simulink model "flexibleBeamSim"  (R2019b)
settings: Solver=ode4  StartTime=0.0  StopTime=tin(end)  FixedStep=Ts  RelTol=1e-3
values from neighbouring files (symbols this model uses):
  shapeit_data =     [GyGzcontroller.mat]    (also in GyGzcontrollerBad.mat; GyGzcontrollerGood.mat; GyGzcontrollerWorse.mat; GzController5Hz.mat)
libraries: cstblocks x1
settings Model: Creator=maxva  LastModifiedBy=maxva

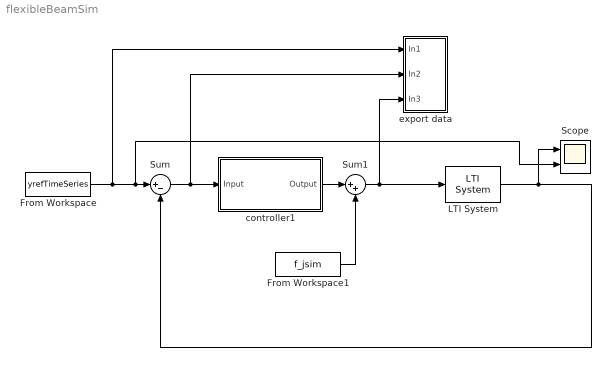
== system flexibleBeamSim ==
  From Workspace : FromWorkspace  VariableName=yrefTimeSeries  SampleTime=0
  From Workspace1 : FromWorkspace  VariableName=f_jsim  SampleTime=0
  LTI System : cstblocks/LTI System  sys=G  IC=[]
  Scope : Scope  NumInputPorts=2
  Sum : Sum  Inputs=|+-
  Sum1 : Sum  Inputs=|++
  controller1 : Subsystem
  export data : Subsystem
  wires:
  LTI System/1 -> Scope/1, Sum/2
  Sum1/1 -> LTI System/1, export data/3(In3)
  From Workspace/1 -> Scope/2, Sum/1, export data/1(In1)
  From Workspace1/1 -> Sum1/2
  Sum/1 -> controller1/1(Input), export data/2(In2)
  controller1/1(Output) -> Sum1/1

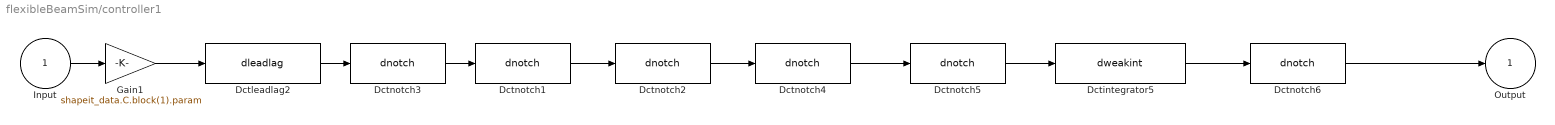
== system flexibleBeamSim/controller1 ==
  Input : Inport
  Dctintegrator5 : S-Function  FunctionName=dweakint  Parameters=f_num, 0.001  SFunctionDeploymentMode=off  EnableBusSupport=off  mask(dctools){f_num=shapeit_data.C.block(8).param}
      mask prompts: f_num "Zero [Hz]"
      mask help: This block implements a discrete time weak integrator filter.
      mask Display: disp('DCT integrator')
  Dctleadlag2 : S-Function  FunctionName=dleadlag  Parameters=f_num, f_den, 0.001  SFunctionDeploymentMode=off  EnableBusSupport=off  mask(dctools){f_num=shapeit_data.C.block(2).param(1), f_den=shapeit_data.C.block(2).param(2)}
      mask prompts: f_num "Zero [Hz]"; f_den "Pole [Hz]"
      mask help: This block implements a discrete time leadlag filter.
      mask Display: disp('DCT leadlag')
  Dctnotch1 : S-Function  FunctionName=dnotch  Parameters=f_num, b_num, f_den, b_den, 0.001  SFunctionDeploymentMode=off  EnableBusSupport=off  mask(dctools){f_num=shapeit_data.C.block(4).param(1), b_num=shapeit_data.C.block(4).param(2), f_den=shapeit_data.C.block(4).param(3), b_den=shapeit_data.C.block(4).param(4)}
      mask prompts: f_num "Zero [Hz]"; b_num "Damping zero [-]"; f_den "Pole [Hz]"; b_den "Damping pole [-]"
      mask help: This block implements a dicrete time 2nd order notch filter.
      mask Display: disp('DCT notch')
  Dctnotch2 : S-Function  FunctionName=dnotch  Parameters=f_num, b_num, f_den, b_den, 0.001  SFunctionDeploymentMode=off  EnableBusSupport=off  mask(dctools){f_num=shapeit_data.C.block(7).param(1), b_num=shapeit_data.C.block(7).param(2), f_den=shapeit_data.C.block(7).param(3), b_den=shapeit_data.C.block(7).param(4)}
      mask prompts: f_num "Zero [Hz]"; b_num "Damping zero [-]"; f_den "Pole [Hz]"; b_den "Damping pole [-]"
      mask help: This block implements a dicrete time 2nd order notch filter.
      mask Display: disp('DCT notch')
  Dctnotch3 : S-Function  FunctionName=dnotch  Parameters=f_num, b_num, f_den, b_den, 0.001  SFunctionDeploymentMode=off  EnableBusSupport=off  mask(dctools){f_num=shapeit_data.C.block(3).param(1), b_num=shapeit_data.C.block(3).param(2), f_den=shapeit_data.C.block(3).param(3), b_den=shapeit_data.C.block(3).param(4)}
      mask prompts: f_num "Zero [Hz]"; b_num "Damping zero [-]"; f_den "Pole [Hz]"; b_den "Damping pole [-]"
      mask help: This block implements a dicrete time 2nd order notch filter.
      mask Display: disp('DCT notch')
  Dctnotch4 : S-Function  FunctionName=dnotch  Parameters=f_num, b_num, f_den, b_den, 0.001  SFunctionDeploymentMode=off  EnableBusSupport=off  mask(dctools){f_num=shapeit_data.C.block(5).param(1), b_num=shapeit_data.C.block(5).param(2), f_den=shapeit_data.C.block(5).param(3), b_den=shapeit_data.C.block(5).param(4)}
      mask prompts: f_num "Zero [Hz]"; b_num "Damping zero [-]"; f_den "Pole [Hz]"; b_den "Damping pole [-]"
      mask help: This block implements a dicrete time 2nd order notch filter.
      mask Display: disp('DCT notch')
  Dctnotch5 : S-Function  FunctionName=dnotch  Parameters=f_num, b_num, f_den, b_den, 0.001  SFunctionDeploymentMode=off  EnableBusSupport=off  mask(dctools){f_num=shapeit_data.C.block(6).param(1), b_num=shapeit_data.C.block(6).param(2), f_den=shapeit_data.C.block(6).param(3), b_den=shapeit_data.C.block(6).param(4)}
      mask prompts: f_num "Zero [Hz]"; b_num "Damping zero [-]"; f_den "Pole [Hz]"; b_den "Damping pole [-]"
      mask help: This block implements a dicrete time 2nd order notch filter.
      mask Display: disp('DCT notch')
  Dctnotch6 : S-Function  FunctionName=dnotch  Parameters=f_num, b_num, f_den, b_den, 0.001  SFunctionDeploymentMode=off  EnableBusSupport=off  mask(dctools){f_num=shapeit_data.C.block(9).param(1), b_num=shapeit_data.C.block(9).param(2), f_den=shapeit_data.C.block(9).param(3), b_den=shapeit_data.C.block(9).param(4)}
      mask prompts: f_num "Zero [Hz]"; b_num "Damping zero [-]"; f_den "Pole [Hz]"; b_den "Damping pole [-]"
      mask help: This block implements a dicrete time 2nd order notch filter.
      mask Display: disp('DCT notch')
  Gain1 : Gain  Gain=shapeit_data.C.block(1).param  SaturateOnIntegerOverflow=on  OutDataTypeStr=Inherit: Same as input  ParamDataTypeStr=Inherit: Same as input
  Output : Outport
  wires:
  Input/1 -> Gain1/1
  Gain1/1 -> Dctleadlag2/1
  Dctleadlag2/1 -> Dctnotch3/1
  Dctnotch3/1 -> Dctnotch1/1
  Dctnotch1/1 -> Dctnotch2/1
  Dctnotch2/1 -> Dctnotch4/1
  Dctnotch4/1 -> Dctnotch5/1
  Dctnotch5/1 -> Dctintegrator5/1
  Dctintegrator5/1 -> Dctnotch6/1
  Dctnotch6/1 -> Output/1

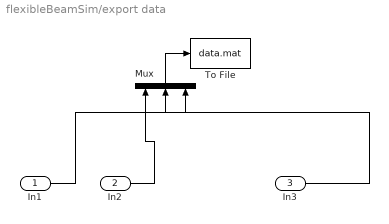
== system flexibleBeamSim/export data ==
  In1 : Inport
  In2 : Inport  Port=2
  In3 : Inport  Port=3
  Mux : Mux  Inputs=3
  To File : ToFile  Filename=data.mat
  wires:
  Mux/1 -> To File/1
  In3/1 -> Mux/2
  In1/1 -> Mux/3
  In2/1 -> Mux/1
